simulink model "NonLinear_Plant_D02"  (R2020b)
settings: Solver=ode3  StartTime=0.0  StopTime=10.0  FixedStep=0.001  RelTol=1e-3
values from neighbouring files (symbols this model uses):
  alpha0 = 180*pi/180    (= 3.14159265359)    [Initialize.m]
  alpha_dot0 = 0    [Initialize.m]
  D_p = 0.0005    [Initialize.m]
  D_r = 0.0015    [Initialize.m]
  g = 9.8    [Initialize.m]
  J_p = 3.4e-5    (= 3.4e-05)    [Initialize.m]
  J_r = 5.7e-5    (= 5.7e-05)    [Initialize.m]
  K_m = 0.042    [Initialize.m]
  L_p = 0.13    [Initialize.m]
  L_r = 0.085    [Initialize.m]
  m_p = 0.024    [Initialize.m]
  R_m = 8.4    [Initialize.m]
  theta0 = 0    [Initialize.m]
  theta_dot0 = 0    [Initialize.m]
undefined symbols (not defined in the file or in its folder): gaussian, K
libraries: simulink x1
settings Model: Creator=Amir  LastModifiedBy=vahed

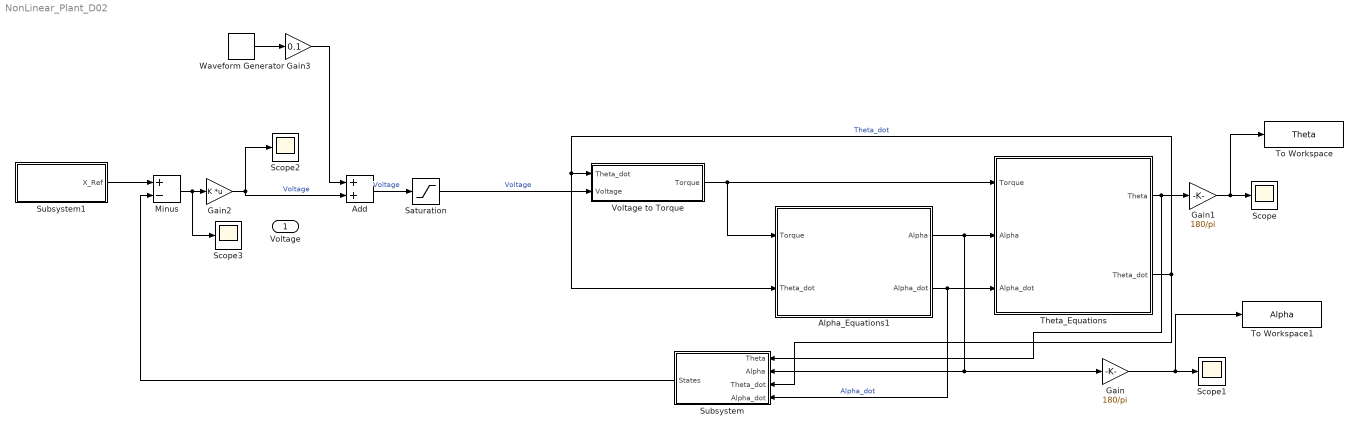
== system NonLinear_Plant_D02 ==
  Voltage : Inport
  Add : Sum
  Alpha_Equations1 : Subsystem
  Gain : Gain  Gain=180/pi
  Gain1 : Gain  Gain=180/pi
  Gain2 : Gain  Gain=K  Multiplication=Matrix(K*u)
  Gain3 : Gain  Gain=0.1
  Minus : Sum  Inputs=+-
  Saturation : Saturate  UpperLimit=15  LowerLimit=-15
  Scope{,1..3} (4 alike) : Scope
  Subsystem : Subsystem
  Subsystem1 : Subsystem
  Theta_Equations : Subsystem
  To Workspace : ToWorkspace  VariableName=Theta  SaveFormat=Timeseries  SampleTime=-1
  To Workspace1 : ToWorkspace  VariableName=Alpha  SaveFormat=Timeseries  SampleTime=-1
  Voltage to Torque : Subsystem
  Waveform Generator : simulink/Sources/Waveform Generator  OutMin=[]  OutMax=[]  OutDataTypeStr=double  SelectedSignal=1  Signals=gaussian('Mean',0,'Variance',1)  BlockNames=MultiportSwitch_429da8b632dd481  SampleTime=0.01
  wires:
  Add/1 -> Saturation/1  "Voltage"
  Theta_Equations/2(Theta_dot) -> Alpha_Equations1/2(Theta_dot), Voltage to Torque/1(Theta_dot), Subsystem/3(Theta_dot)  "Theta_dot"
  Voltage to Torque/1(Torque) -> Alpha_Equations1/1(Torque), Theta_Equations/1(Torque)
  Theta_Equations/1(Theta) -> Subsystem/1(Theta), Gain1/1
  Gain/1 -> To Workspace1/1, Scope1/1
  Alpha_Equations1/1(Alpha) -> Gain/1, Subsystem/2(Alpha), Theta_Equations/2(Alpha)
  Alpha_Equations1/2(Alpha_dot) -> Theta_Equations/3(Alpha_dot), Subsystem/4(Alpha_dot)  "Alpha_dot"
  Gain1/1 -> To Workspace/1, Scope/1
  Gain2/1 -> Add/2, Scope2/1  "Voltage"
  Subsystem1/1(X_Ref) -> Minus/1
  Subsystem/1(States) -> Minus/2
  Minus/1 -> Scope3/1, Gain2/1
  Waveform Generator/1 -> Gain3/1
  Gain3/1 -> Add/1
  Saturation/1 -> Voltage to Torque/2(Voltage)  "Voltage"

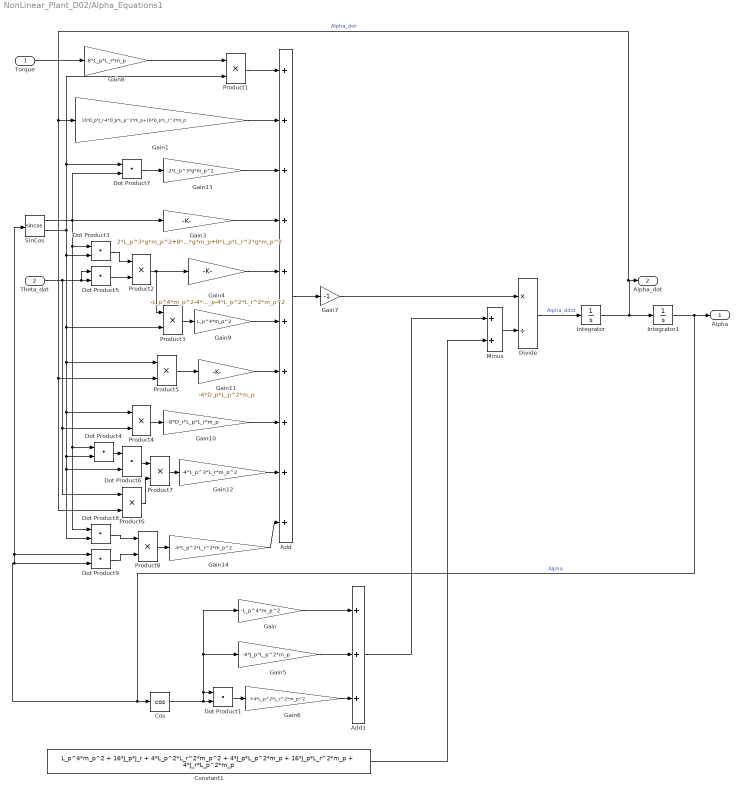
== system NonLinear_Plant_D02/Alpha_Equations1 ==
  Torque : Inport
  Theta_dot : Inport  Port=2
  Add : Sum  Inputs=++++++++++
  Add1 : Sum  Inputs=+++
  Constant1 : Constant  Value=L_p^4*m_p^2 + 16*J_p*J_r + 4*L_p^2*L_r^2*m_p^2 + 4*J_p*L_p^2*m_p + 16*J_p*L_r^2*m_p + 4*J_r*L_p^2*m_p
  Cos : Trigonometry  Operator=cos
  Divide : Product  Inputs=*/
  Dot Product{1,3..9} (8 alike) : DotProduct  InputSameDT=on  OutDataTypeStr=Inherit: Inherit via internal rule
  Gain : Gain  Gain=-L_p^4*m_p^2
  Gain1 : Gain  Gain=16*D_p*J_r-4*D_p*L_p^2*m_p+16*D_p*L_r^2*m_p
  Gain10 : Gain  Gain=-8*D_r*L_p*L_r*m_p
  Gain11 : Gain  Gain=-4*D_p*L_p^2*m_p
  Gain12 : Gain  Gain=-4*L_p^3*L_r*m_p^2
  Gain13 : Gain  Gain=-2*L_p^3*g*m_p^2
  Gain14 : Gain  Gain=-4*L_p^2*L_r^2*m_p^2
  Gain3 : Gain  Gain=2*L_p^3*g*m_p^2+8*J_r*L_p*g*m_p+8*L_p*L_r^2*g*m_p^2
  Gain4 : Gain  Gain=-L_p^4*m_p^2-4*J_r*L_p^2*m_p-4*L_p^2*L_r^2*m_p^2
  Gain5 : Gain  Gain=-4*J_p*L_p^2*m_p
  Gain6 : Gain  Gain=+4*L_p^2*L_r^2*m_p^2
  Gain7 : Gain  Gain=-1
  Gain8 : Gain  Gain=8*L_p*L_r*m_p
  Gain9 : Gain  Gain=L_p^4*m_p^2
  Integrator : Integrator  InitialCondition=alpha_dot0
  Integrator1 : Integrator  InitialCondition=alpha0
  Minus : Sum
  Product{1..8} (8 alike) : Product
  SinCos : Trigonometry  Operator=sincos
  Alpha : Outport
  Alpha_dot : Outport  Port=2
  wires:
  Theta_dot/1 -> Dot Product5/1, Dot Product5/2, Product6/1, Product4/2
  Gain3/1 -> Add/4
  SinCos/1 -> Gain3/1, Dot Product7/2, Dot Product3/1, Dot Product8/1, Dot Product4/1
  Gain13/1 -> Add/3
  Gain1/1 -> Add/2
  Gain8/1 -> Product1/1
  Add/1 -> Gain7/1
  Add1/1 -> Minus/1
  Gain/1 -> Add1/1
  Gain5/1 -> Add1/2
  Gain6/1 -> Add1/3
  Dot Product1/1 -> Gain6/1
  Cos/1 -> Dot Product1/2, Gain/1, Gain5/1, Dot Product1/1
  Torque/1 -> Gain8/1
  Minus/1 -> Divide/2
  Constant1/1 -> Minus/2
  Divide/1 -> Integrator/1  "Alpha_ddot"
  Integrator/1 -> Alpha_dot/1, Gain1/1, Product5/2, Product6/2, Integrator1/1  "Alpha_dot"
  Integrator1/1 -> Cos/1, Dot Product9/2, Dot Product9/1, SinCos/1, Alpha/1  "Alpha"
  Gain7/1 -> Divide/1
  Product1/1 -> Add/1
  Dot Product5/1 -> Product2/2
  Dot Product3/1 -> Product2/1
  Product2/1 -> Product3/1, Gain4/1
  Gain4/1 -> Add/5
  Gain9/1 -> Add/6
  Product3/1 -> Gain9/1
  SinCos/2 -> Product1/2, Dot Product7/1, Product5/1, Dot Product8/2, Dot Product6/2, Dot Product4/2, Product4/1, Product3/2, Dot Product3/2
  Product4/1 -> Gain10/1
  Gain10/1 -> Add/8
  Gain11/1 -> Add/7
  Product5/1 -> Gain11/1
  Dot Product4/1 -> Dot Product6/1
  Dot Product6/1 -> Product7/1
  Product6/1 -> Product7/2
  Product7/1 -> Gain12/1
  Gain12/1 -> Add/9
  Dot Product7/1 -> Gain13/1
  Gain14/1 -> Add/10
  Product8/1 -> Gain14/1
  Dot Product8/1 -> Product8/1
  Dot Product9/1 -> Product8/2

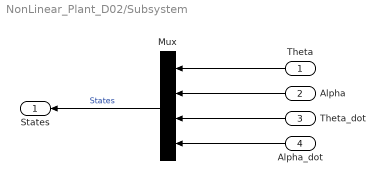
== system NonLinear_Plant_D02/Subsystem ==
  Theta : Inport
  Alpha : Inport  Port=2
  Theta_dot : Inport  Port=3
  Alpha_dot : Inport  Port=4
  Mux : Mux
  States : Outport
  wires:
  Alpha_dot/1 -> Mux/4
  Mux/1 -> States/1  "States"
  Theta_dot/1 -> Mux/3
  Theta/1 -> Mux/1
  Alpha/1 -> Mux/2

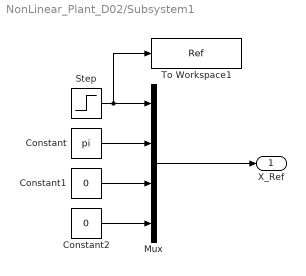
== system NonLinear_Plant_D02/Subsystem1 ==
  Constant : Constant  Value=pi
  Constant1 : Constant  Value=0
  Constant2 : Constant  Value=0
  Mux : Mux
  Step : Step  Time=2  After=pi/2  SampleTime=0
  To Workspace1 : ToWorkspace  VariableName=Ref  SaveFormat=Timeseries  SampleTime=-1
  X_Ref : Outport
  wires:
  Mux/1 -> X_Ref/1
  Constant/1 -> Mux/2
  Constant2/1 -> Mux/4
  Constant1/1 -> Mux/3
  Step/1 -> To Workspace1/1, Mux/1

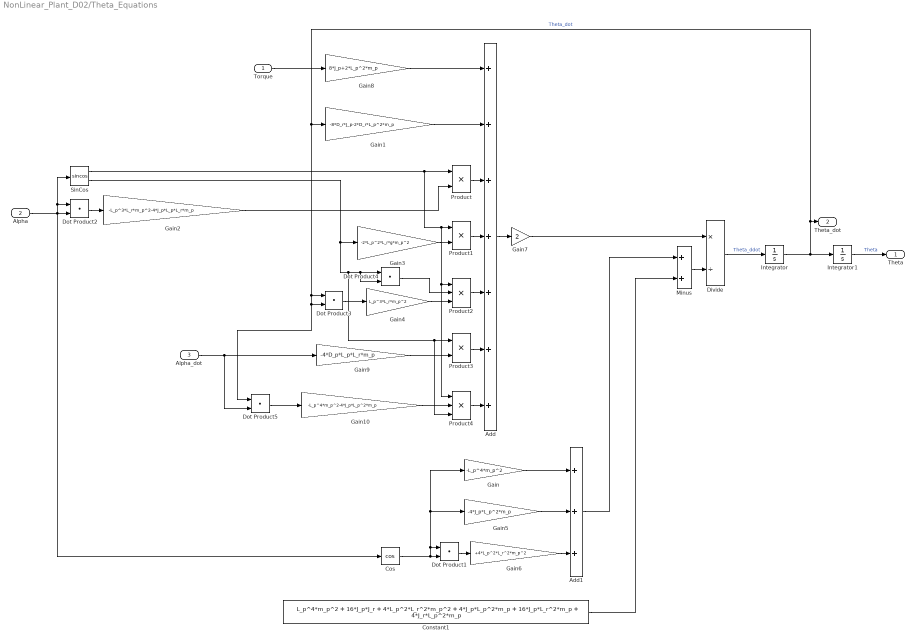
== system NonLinear_Plant_D02/Theta_Equations ==
  Torque : Inport
  Alpha : Inport  Port=2
  Alpha_dot : Inport  Port=3
  Add : Sum  Inputs=+++++++
  Add1 : Sum  Inputs=+++
  Constant1 : Constant  Value=L_p^4*m_p^2 + 16*J_p*J_r + 4*L_p^2*L_r^2*m_p^2 + 4*J_p*L_p^2*m_p + 16*J_p*L_r^2*m_p + 4*J_r*L_p^2*m_p
  Cos : Trigonometry  Operator=cos
  Divide : Product  Inputs=*/
  Dot Product{1..5} (5 alike) : DotProduct  InputSameDT=on  OutDataTypeStr=Inherit: Inherit via internal rule
  Gain : Gain  Gain=-L_p^4*m_p^2
  Gain1 : Gain  Gain=-8*D_r*J_p-2*D_r*L_p^2*m_p
  Gain10 : Gain  Gain=-L_p^4*m_p^2-4*J_p*L_p^2*m_p
  Gain2 : Gain  Gain=-L_p^3*L_r*m_p^2-4*J_p*L_p*L_r*m_p
  Gain3 : Gain  Gain=-2*L_p^2*L_r*g*m_p^2
  Gain4 : Gain  Gain=L_p^3*L_r*m_p^2
  Gain5 : Gain  Gain=-4*J_p*L_p^2*m_p
  Gain6 : Gain  Gain=+4*L_p^2*L_r^2*m_p^2
  Gain7 : Gain  Gain=2
  Gain8 : Gain  Gain=8*J_p+2*L_p^2*m_p
  Gain9 : Gain  Gain=-4*D_p*L_p*L_r*m_p
  Integrator : Integrator  InitialCondition=theta_dot0
  Integrator1 : Integrator  InitialCondition=theta0
  Minus : Sum
  Product : Product
  Product1 : Product
  Product2 : Product  Inputs=3
  Product3 : Product
  Product4 : Product  Inputs=3
  SinCos : Trigonometry  Operator=sincos
  Theta : Outport
  Theta_dot : Outport  Port=2
  wires:
  Add/1 -> Gain7/1
  Integrator1/1 -> Theta/1  "Theta"
  Integrator/1 -> Integrator1/1, Dot Product5/1, Dot Product3/2, Dot Product3/1, Gain1/1, Theta_dot/1  "Theta_dot"
  Divide/1 -> Integrator/1  "Theta_ddot"
  Constant1/1 -> Minus/2
  Minus/1 -> Divide/2
  Torque/1 -> Gain8/1
  Cos/1 -> Dot Product1/1, Gain5/1, Gain/1, Dot Product1/2
  Dot Product1/1 -> Gain6/1
  Gain6/1 -> Add1/3
  Gain5/1 -> Add1/2
  Gain/1 -> Add1/1
  Add1/1 -> Minus/1
  Gain7/1 -> Divide/1
  Gain8/1 -> Add/1
  Gain1/1 -> Add/2
  Alpha/1 -> Cos/1, SinCos/1, Dot Product2/1, Dot Product2/2
  Product/1 -> Add/3
  SinCos/1 -> Product4/1, Product2/1, Product1/1, Product/1
  Dot Product2/1 -> Gain2/1
  Gain2/1 -> Product/2
  Product1/1 -> Add/4
  Gain3/1 -> Product1/2
  Product2/1 -> Add/5
  Dot Product3/1 -> Gain4/1
  SinCos/2 -> Product4/3, Product3/1, Dot Product4/2, Dot Product4/1, Gain3/1
  Dot Product4/1 -> Product2/2
  Gain4/1 -> Product2/3
  Product3/1 -> Add/6
  Alpha_dot/1 -> Dot Product5/2, Gain9/1
  Gain9/1 -> Product3/2
  Dot Product5/1 -> Gain10/1
  Product4/1 -> Add/7
  Gain10/1 -> Product4/2

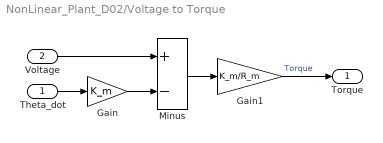
== system NonLinear_Plant_D02/Voltage to Torque ==
  Theta_dot : Inport
  Voltage : Inport  Port=2
  Gain : Gain  Gain=K_m
  Gain1 : Gain  Gain=K_m/R_m
  Minus : Sum  Inputs=+-
  Torque : Outport
  wires:
  Gain/1 -> Minus/2
  Voltage/1 -> Minus/1
  Gain1/1 -> Torque/1  "Torque"
  Minus/1 -> Gain1/1
  Theta_dot/1 -> Gain/1
